simulink model "RB_KAIROS_ImpControl_OpSpace_quat_2020b_safety"  (R2020b)
settings: Solver=ode4  StartTime=0.0  StopTime=20  FixedStep=model_sample_time  RelTol=1e-3
values from neighbouring files (symbols this model uses):
  am = 0.3    [RB_KAIROS_ImpControl_OpSpace_quat_2020b_safety_main.m]
  am_r = 0.3    [RB_KAIROS_ImpControl_OpSpace_quat_2020b_safety_main.m]
  Kc = diag(50*ones(6,1))    [RB_KAIROS_ImpControl_OpSpace_quat_2020b_safety_main.m]
  Kp = 2*[400;400;400;400;0;0;0]    [RB_KAIROS_ImpControl_OpSpace_quat_2020b_safety_main.m]
  Kv = [1000;1000;1000;[300;300;300;300;300;300;300]]    [RB_KAIROS_ImpControl_OpSpace_quat_2020b_safety_main.m]
  model_sample_time = 0.001    [RB_KAIROS_ImpControl_OpSpace_quat_2020b_safety_main.m]
  q_dot_0 = zeros(10,1)    [RB_KAIROS_ImpControl_OpSpace_quat_2020b_safety_main.m]
  T_i = K    [RB_KAIROS_ImpControl_OpSpace_quat_2020b_safety_main.m]
  tau_ext = [0 0 0 0 0 0 0 0 0 0 0]    [RB_KAIROS_ImpControl_OpSpace_quat_2020b_safety_main.m]
  v_SMU = 10    [RB_KAIROS_ImpControl_OpSpace_quat_2020b_safety_main.m]
  vm = 0.5    [RB_KAIROS_ImpControl_OpSpace_quat_2020b_safety_main.m]
  vm_r = 0.5    [RB_KAIROS_ImpControl_OpSpace_quat_2020b_safety_main.m]
undefined symbols (not defined in the file or in its folder): DiscIntNeverNeededParam, magnitude, q_0, sigbuilder_block, T_f
libraries: simulink x4, utils x4, transformations_lib x3
(part 1 of 17)
settings Model: Creator=Alessandro  LastModifiedBy=ubuntu
settings DataIOCC: ReturnWorkspaceOutputs=off
settings DebuggingCC: UnconnectedInputMsg=none  UnconnectedOutputMsg=none  UnconnectedLineMsg=none  SFMachineParentedDataDiag=error
settings SFSimCC: SimUserIncludeDirs="\"/home/ubuntu/whole_body_control/whole-body-controller/Simulation/GeneratedFunctions/CppDynamics/include\""  SimTargetLang=C++
settings SFSimCC: SimCustomHeaderCode=|
  | #include "get_C.h"
  | #include "get_Cv.h"
  | #include "get_M.h"
  | #include "get_Mv.h"
  | #include "get_G.h"
settings SFSimCC: SimUserSources=|
  | "/home/ubuntu/whole_body_control/whole-body-controller/Simulation/GeneratedFunctions/CppDynamics/src/get_C.cpp"
  | "/home/ubuntu/whole_body_control/whole-body-controller/Simulation/GeneratedFunctions/CppDynamics/src/get_Cv.cpp"
  | "/home/ubuntu/whole_body_control/whole-body-controller/Simulation/GeneratedFunctions/CppDynamics/src/get_M.cpp"
  | "/home/ubuntu/whole_body_control/whole-body-controller/Simulation/GeneratedFunctions/CppDynamics/src/get_Mv.cpp"
  | "/home/ubuntu/whole_body_control/whole-body-controller/Simulation/GeneratedFunctions/CppDynamics/src/get_G.cpp"

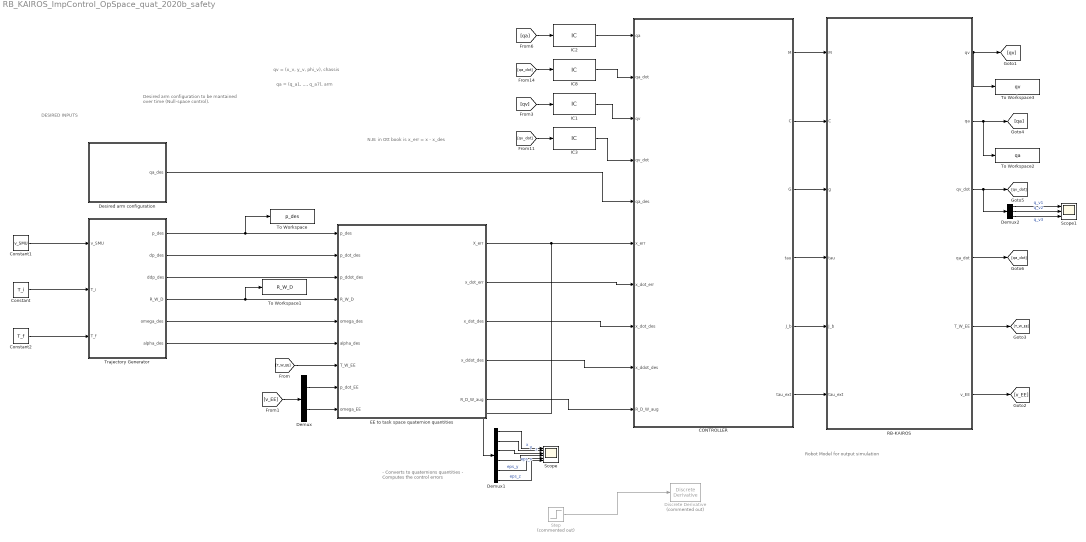
== system RB_KAIROS_ImpControl_OpSpace_quat_2020b_safety ==
  note: - Converts to quaternions quantities
      | - Computes the control errors
  note: Robot Model for output simulation
  note: DESIRED INPUTS
  note: N.B: in Ott book is x_err = x - x_des
  note: qv = (x_v, y_v, phi_v), chassis
  note: qa = (q_a1, ..., q_a7), arm
  note: Desired arm configuration to be mantained over time (Null-space control).
  "CONTROLLER " : Subsystem
  Constant : Constant  Value=T_i
  Constant1 : Constant  Value=v_SMU
  Constant2 : Constant  Value=T_f
  Demux : Demux  Outputs=2
  Demux1 : Demux  Outputs=6
  Demux2 : Demux  Outputs=3
  Desired arm configuration : Subsystem
  Discrete Derivative : simulink/Discrete/Discrete Derivative  Commented=on  gainval=1  ICPrevScaledInput=0.0  OutMin=[]  OutMax=[]  OutDataType=fixdt(1, 16)  OutScaling=2^-10  DoSatur=off
  EE to task space quaternion quantities : Subsystem
  IC1 : InitialCondition  Value=q_0([1:3])
  IC2 : InitialCondition  Value=q_0([4:10])
  IC3 : InitialCondition  Value=q_dot_0([1:3])
  IC8 : InitialCondition  Value=q_dot_0([4:10])
  RB-KAIROS : Subsystem
  Scope : Scope  NumInputPorts=6
  Scope1 : Scope  NumInputPorts=3
  Step : Step  Commented=on  Time=5  Before=zeros(10,1)  After=tau_ext  SampleTime=0
  To Workspace : ToWorkspace  VariableName=p_des  SaveFormat=Timeseries  SampleTime=-1
  To Workspace1 : ToWorkspace  VariableName=R_W_D  SaveFormat=Timeseries  SampleTime=-1
  To Workspace2 : ToWorkspace  VariableName=qa  SaveFormat=Timeseries  SampleTime=-1
      settings: Decimation=10
  To Workspace3 : ToWorkspace  VariableName=qv  SaveFormat=Timeseries  SampleTime=-1
      settings: Decimation=10
  Trajectory Generator : Subsystem
  wires:
  "CONTROLLER "/1(M) -> RB-KAIROS/1(M)
  RB-KAIROS/4(qa_dot) -> [qa_dot]
  RB-KAIROS/6(v_EE) -> [v_EE]
  "CONTROLLER "/3(G) -> RB-KAIROS/3(g)
  RB-KAIROS/2(qa) -> [qa], To Workspace2/1
  [qa_dot] -> IC8/1
  Desired arm configuration/1(qa_des) -> "CONTROLLER "/5(qa_des)
  [qv] -> IC1/1
  "CONTROLLER "/2(C) -> RB-KAIROS/2(C)
  RB-KAIROS/5(T_W_EE) -> [T_W_EE]
  [qv_dot] -> IC3/1
  "CONTROLLER "/4(tau) -> RB-KAIROS/4(tau)
  [qa] -> IC2/1
  RB-KAIROS/1(qv) -> [qv], To Workspace3/1
  [T_W_EE] -> EE to task space quaternion quantities/7(T_W_EE)
  "CONTROLLER "/5(J_b) -> RB-KAIROS/5(J_b)
  [v_EE] -> Demux/1
  Demux/2 -> EE to task space quaternion quantities/9(omega_EE)
  Demux/1 -> EE to task space quaternion quantities/8(p_dot_EE)
  EE to task space quaternion quantities/2(x_dot_err) -> "CONTROLLER "/7(x_dot_err)
  EE to task space quaternion quantities/3(x_dot_des) -> "CONTROLLER "/8(x_dot_des)
  EE to task space quaternion quantities/4(x_ddot_des) -> "CONTROLLER "/9(x_ddot_des)
  EE to task space quaternion quantities/5(R_D_W_aug) -> "CONTROLLER "/10(R_D_W_aug)
  IC2/1 -> "CONTROLLER "/1(qa)
  IC8/1 -> "CONTROLLER "/2(qa_dot)
  IC1/1 -> "CONTROLLER "/3(qv)
  IC3/1 -> "CONTROLLER "/4(qv_dot)
  Constant1/1 -> Trajectory Generator/1(v_SMU)
  Constant/1 -> Trajectory Generator/2(T_i)
  Constant2/1 -> Trajectory Generator/3(T_f)
  Trajectory Generator/1(p_des) -> To Workspace/1, EE to task space quaternion quantities/1(p_des)
  Trajectory Generator/2(dp_des) -> EE to task space quaternion quantities/2(p_dot_des)
  Trajectory Generator/3(ddp_des) -> EE to task space quaternion quantities/3(p_ddot_des)
  Trajectory Generator/5(omega_des) -> EE to task space quaternion quantities/5(omega_des)
  Trajectory Generator/6(alpha_des) -> EE to task space quaternion quantities/6(alpha_des)
  Trajectory Generator/4(R_W_D) -> To Workspace1/1, EE to task space quaternion quantities/4(R_W_D)
  EE to task space quaternion quantities/1(X_err) -> Demux1/1, "CONTROLLER "/6(x_err)
  Demux1/6 -> Scope/6  "eps_z"
  Demux1/4 -> Scope/4  "eps_x"
  Demux1/2 -> Scope/2  "y"
  Demux1/5 -> Scope/5  "eps_y"
  Demux1/3 -> Scope/3  "z"
  Demux1/1 -> Scope/1  "x"
  Demux2/3 -> Scope1/3  "q_v3"
  RB-KAIROS/3(qv_dot) -> Demux2/1, [qv_dot]
  Demux2/2 -> Scope1/2  "q_v2"
  Demux2/1 -> Scope1/1  "q_v1"
  Step/1 -> Discrete Derivative/1
  "CONTROLLER "/6(tau_ext) -> RB-KAIROS/6(tau_ext)

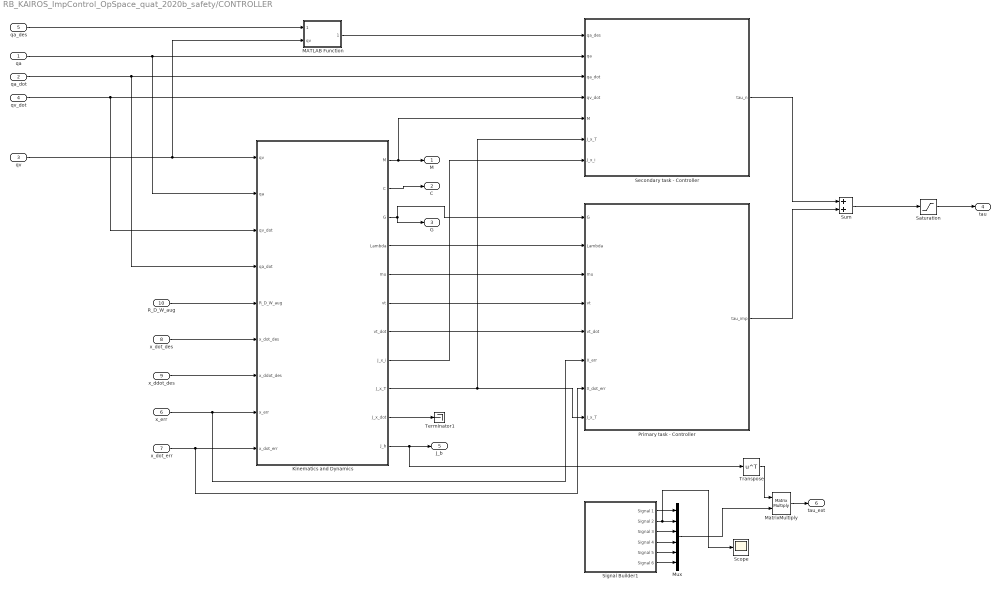
== system RB_KAIROS_ImpControl_OpSpace_quat_2020b_safety/CONTROLLER  ==
  qa : Inport
  qa_dot : Inport  Port=2
  qv : Inport  Port=3
  qv_dot : Inport  Port=4
  qa_des : Inport  Port=5
  x_err : Inport  Port=6
  x_dot_err : Inport  Port=7
  x_dot_des : Inport  Port=8
  x_ddot_des : Inport  Port=9
  R_D_W_aug : Inport  Port=10
  Kinematics and Dynamics : Subsystem
  MATLAB Function : MATLAB Function  TreatAsAtomicUnit=on
  MatrixMultiply : Product  Multiplication=Matrix(*)
  Mux : Mux  Inputs=6
  Primary task - Controller : Subsystem
  Saturation : Saturate  UpperLimit=|  LowerLimit=|
      UpperLimit=|
      | [[300; 300; 300]; 87;
      | 87;
      | 87;
      | 87;
      | 12;
      | 12; 12]
      LowerLimit=|
      | -[[300; 300; 300]; 87;
      | 87;
      | 87;
      | 87;
      | 12;
      | 12; 12]
  Scope : Scope
  Secondary task - Controller : Subsystem
  Signal Builder1 : Subsystem  Tag=STV Subsys  LoadFcn=sigbuilder_block('load',[721.5 -243.75 1378.5 558.75 ]);  StartFcn=sigbuilder_block('start');  StopFcn=sigbuilder_block('stop');  ClipboardFcn=sigbuilder_block('clipboard');  mask(Sigbuilder block){tuvar=[0:10]}
      mask help: Simulink:masks:SigbuilderBlock_MD
      mask init:
      | if ~strcmp(get_param(bdroot(gcbh),'SimulationStatus'),'stopped') tuvar = sigbuilder_block('maskInit'); end
      settings: CopyFcn=sigbuilder_block('copy');  DeleteFcn=sigbuilder_block('delete');  ModelCloseFcn=sigbuilder_block('modelClose');  PreSaveFcn=sigbuilder_block('preSave');  PauseFcn=sigbuilder_block('pause');  ContinueFcn=sigbuilder_block('continue');  NameChangeFcn=sigbuilder_block('namechange');  OpenFcn=sigbuilder_block('open',[-114 -87.75 1386 594 ]);  CloseFcn=sigbuilder_block('close');
      mask Display: plot(0, 0, 100, 100,[2, 2, 32, 32, 2], [68, 8, 8, 68, 68],[32, 2], [38, 38], [32, 19, 2],[53, 60, 44], [32, 17, 17, 2],[16, 16, 31, 31]);txt = getActiveGroup(gcbh);text(2, 100, txt,'verticalAlignment', 'top');
  Sum : Sum
  Terminator1 : Terminator
  Transpose : Math  Operator=transpose  SaturateOnIntegerOverflow=on
  M : Outport
  C : Outport  Port=2
  G : Outport  Port=3
  tau : Outport  Port=4
  J_b : Outport  Port=5
  tau_ext : Outport  Port=6
  wires:
  qv_dot/1 -> Secondary task - Controller/4(qv_dot), Kinematics and Dynamics/3(qv_dot)
  Primary task - Controller/1(tau_imp) -> Sum/2
  qv/1 -> Kinematics and Dynamics/1(qv), MATLAB Function/2(qv)
  qa/1 -> Secondary task - Controller/2(qa), Kinematics and Dynamics/2(qa)
  qa_dot/1 -> Kinematics and Dynamics/4(qa_dot), Secondary task - Controller/3(qa_dot)
  Kinematics and Dynamics/9(J_x_T) -> Primary task - Controller/8(J_x_T), Secondary task - Controller/6(J_x_T)
  Kinematics and Dynamics/8(J_x_i) -> Secondary task - Controller/7(J_x_i)
  Secondary task - Controller/1(tau_n) -> Sum/1
  Kinematics and Dynamics/3(G) -> Primary task - Controller/1(G), G/1
  Sum/1 -> Saturation/1
  Kinematics and Dynamics/1(M) -> M/1, Secondary task - Controller/5(M)
  qa_des/1 -> MATLAB Function/1(qa_des)
  Kinematics and Dynamics/2(C) -> C/1
  Saturation/1 -> tau/1
  R_D_W_aug/1 -> Kinematics and Dynamics/5(R_D_W_aug)
  x_dot_des/1 -> Kinematics and Dynamics/6(x_dot_des)
  x_ddot_des/1 -> Kinematics and Dynamics/7(x_ddot_des)
  x_dot_err/1 -> Primary task - Controller/7(X_dot_err), Kinematics and Dynamics/9(x_dot_err)
  Kinematics and Dynamics/6(vt) -> Primary task - Controller/4(vt)
  Kinematics and Dynamics/7(vt_dot) -> Primary task - Controller/5(vt_dot)
  Kinematics and Dynamics/11(J_b) -> Transpose/1, J_b/1
  Kinematics and Dynamics/10(J_x_dot) -> Terminator1/1
  Kinematics and Dynamics/4(Lambda) -> Primary task - Controller/2(Lambda)
  Kinematics and Dynamics/5(mu) -> Primary task - Controller/3(mu)
  MATLAB Function/1(qa_des_new) -> Secondary task - Controller/1(qa_des)
  x_err/1 -> Kinematics and Dynamics/8(x_err), Primary task - Controller/6(X_err)
  MatrixMultiply/1 -> tau_ext/1
  Transpose/1 -> MatrixMultiply/1
  Mux/1 -> MatrixMultiply/2
  Signal Builder1/5(Signal 5) -> Mux/5
  Signal Builder1/1(Signal 1) -> Mux/1
  Signal Builder1/3(Signal 3) -> Mux/3
  Signal Builder1/6(Signal 6) -> Mux/6
  Signal Builder1/4(Signal 4) -> Mux/4
  Signal Builder1/2(Signal 2) -> Scope/1, Mux/2

== system RB_KAIROS_ImpControl_OpSpace_quat_2020b_safety/Desired arm configuration ==
  Constant : Constant  Value=[0, -0.785, 0, -2.356, 0, 1.57, 0.785]'  SampleTime=model_sample_time
  qa_des : Outport
  wires:
  Constant/1 -> qa_des/1

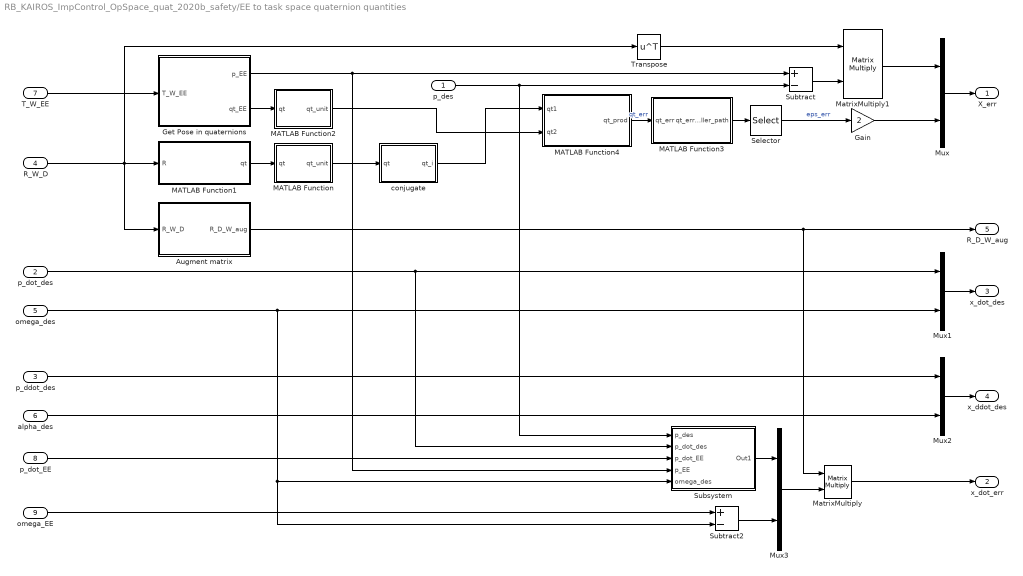
== system RB_KAIROS_ImpControl_OpSpace_quat_2020b_safety/EE to task space quaternion quantities ==
  p_des : Inport
  p_dot_des : Inport  Port=2
  p_ddot_des : Inport  Port=3
  R_W_D : Inport  Port=4
  omega_des : Inport  Port=5
  alpha_des : Inport  Port=6
  T_W_EE : Inport  Port=7
  p_dot_EE : Inport  Port=8
  omega_EE : Inport  Port=9
  Augment matrix : MATLAB Function  TreatAsAtomicUnit=on
  Gain : Gain  Gain=2
  Get Pose in quaternions : MATLAB Function  TreatAsAtomicUnit=on
  MATLAB Function : MATLAB Function  TreatAsAtomicUnit=on
  MATLAB Function1 : MATLAB Function  TreatAsAtomicUnit=on
  MATLAB Function2 : MATLAB Function  TreatAsAtomicUnit=on
  MATLAB Function3 : MATLAB Function  TreatAsAtomicUnit=on
  MATLAB Function4 : MATLAB Function  TreatAsAtomicUnit=on
  MatrixMultiply : Product  Multiplication=Matrix(*)
  MatrixMultiply1 : Product  Multiplication=Matrix(*)
  Mux{,1..3} (4 alike) : Mux  Inputs=2
  Selector : Selector  InputPortWidth=4  IndexOptions=Index vector (dialog)  Indices=[2:4]  OutputSizes=1
  Subsystem : Subsystem
  Subtract : Sum  Inputs=+-
  Subtract2 : Sum  Inputs=+-
  Transpose : Math  Operator=transpose  SaturateOnIntegerOverflow=on
  conjugate : MATLAB Function  TreatAsAtomicUnit=on
  X_err : Outport
  x_dot_err : Outport  Port=2
  x_dot_des : Outport  Port=3
  x_ddot_des : Outport  Port=4
  R_D_W_aug : Outport  Port=5
  wires:
  Get Pose in quaternions/1(p_EE) -> Subtract/1, Subsystem/4(p_EE)
  Subtract/1 -> MatrixMultiply1/2
  p_des/1 -> Subtract/2, Subsystem/1(p_des)
  T_W_EE/1 -> Get Pose in quaternions/1(T_W_EE)
  MATLAB Function4/1(qt_prod) -> MATLAB Function3/1(qt_err)  "qt_err"
  R_W_D/1 -> MATLAB Function1/1(R), Transpose/1, Augment matrix/1(R_W_D)
  Mux/1 -> X_err/1
  MATLAB Function1/1(qt) -> MATLAB Function/1(qt)
  p_dot_des/1 -> Mux1/1, Subsystem/2(p_dot_des)
  Get Pose in quaternions/2(qt_EE) -> MATLAB Function2/1(qt)
  Selector/1 -> Gain/1  "eps_err"
  Augment matrix/1(R_D_W_aug) -> R_D_W_aug/1, MatrixMultiply/1
  omega_des/1 -> Mux1/2, Subsystem/5(omega_des), Subtract2/2
  Mux1/1 -> x_dot_des/1
  Mux2/1 -> x_ddot_des/1
  alpha_des/1 -> Mux2/2
  p_ddot_des/1 -> Mux2/1
  omega_EE/1 -> Subtract2/1
  Subtract2/1 -> Mux3/2
  Mux3/1 -> MatrixMultiply/2
  MatrixMultiply/1 -> x_dot_err/1
  MatrixMultiply1/1 -> Mux/1
  Gain/1 -> Mux/2
  p_dot_EE/1 -> Subsystem/3(p_dot_EE)
  Subsystem/1(Out1) -> Mux3/1
  MATLAB Function/1(qt_unit) -> conjugate/1(qt)
  MATLAB Function2/1(qt_unit) -> MATLAB Function4/2(qt2)
  conjugate/1(qt_i) -> MATLAB Function4/1(qt1)
  Transpose/1 -> MatrixMultiply1/1
  MATLAB Function3/1(qt_err_smaller_path) -> Selector/1

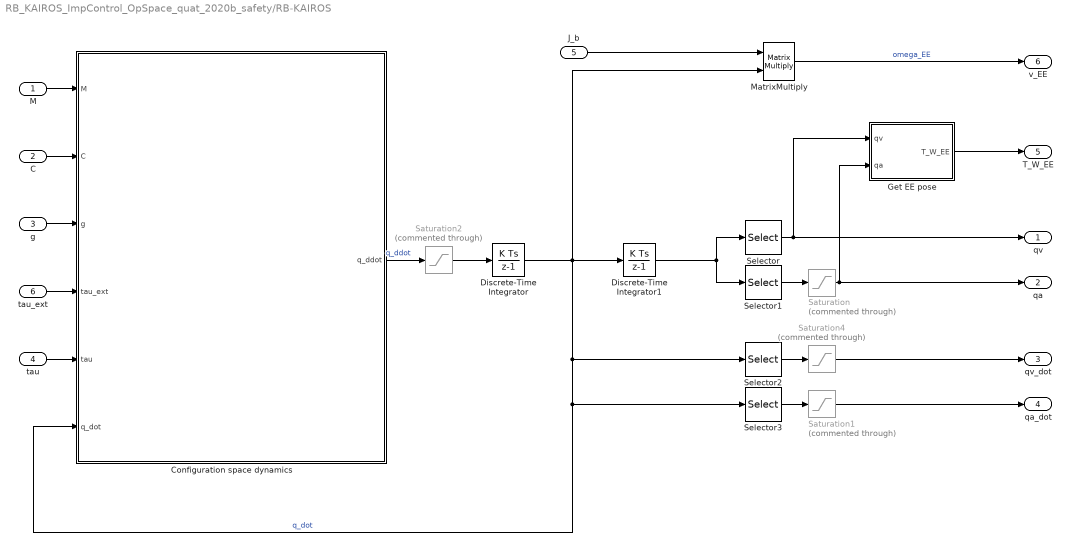
== system RB_KAIROS_ImpControl_OpSpace_quat_2020b_safety/RB-KAIROS ==
  M : Inport
  C : Inport  Port=2
  g : Inport  Port=3
  tau : Inport  Port=4
  J_b : Inport  Port=5
  tau_ext : Inport  Port=6
  Configuration space dynamics : MATLAB Function  TreatAsAtomicUnit=on
  Discrete-Time Integrator : DiscreteIntegrator  InitialCondition=q_dot_0  SampleTime=model_sample_time  ICPrevOutput=DiscIntNeverNeededParam  ICPrevScaledInput=DiscIntNeverNeededParam
  Discrete-Time Integrator1 : DiscreteIntegrator  InitialCondition=q_0  SampleTime=model_sample_time  ICPrevOutput=DiscIntNeverNeededParam  ICPrevScaledInput=DiscIntNeverNeededParam
  Get EE pose : Subsystem
  MatrixMultiply : Product  Multiplication=Matrix(*)
  Saturation : Saturate  Commented=through  UpperLimit=[2.3093; 1.5133; 2.4937; -0.4461; 2.4800; 4.2094; 2.6895]  LowerLimit=[-2.3093; -1.5133; -2.4937; -2.7478; -2.4800; 0.8521; -2.6895]
  Saturation1 : Saturate  Commented=through  UpperLimit=[2; 1; 1.5; 1.25; 3; 1.5; 3]  LowerLimit=-[2; 1; 1.5; 1.25; 3; 1.5; 3]
  Saturation2 : Saturate  Commented=through  UpperLimit=|  LowerLimit=|
      UpperLimit=|
      | [20*ones(3,1); 15;
      | 7.5;
      | 10;
      | 12.5;
      | 15;
      | 20;
      | 20;]
      LowerLimit=|
      | -[20*ones(3,1); 15;
      | 7.5;
      | 10;
      | 12.5;
      | 15;
      | 20;
      | 20;]
  Saturation4 : Saturate  Commented=through  UpperLimit=1*ones(3,1)  LowerLimit=-1*ones(3,1)
  Selector : Selector  IndexOptions=Index vector (dialog)  Indices=[1:3]  OutputSizes=1
  Selector1 : Selector  IndexOptions=Index vector (dialog)  Indices=[4:10]  OutputSizes=1
  Selector2 : Selector  IndexOptions=Index vector (dialog)  Indices=[1:3]  OutputSizes=1
  Selector3 : Selector  IndexOptions=Index vector (dialog)  Indices=[4:10]  OutputSizes=1
  qv : Outport
  qa : Outport  Port=2
  qv_dot : Outport  Port=3
  qa_dot : Outport  Port=4
  T_W_EE : Outport  Port=5
  v_EE : Outport  Port=6
  wires:
  M/1 -> Configuration space dynamics/1(M)
  C/1 -> Configuration space dynamics/2(C)
  g/1 -> Configuration space dynamics/3(g)
  tau/1 -> Configuration space dynamics/5(tau)
  tau_ext/1 -> Configuration space dynamics/4(tau_ext)
  Configuration space dynamics/1(q_ddot) -> Saturation2/1  "q_ddot"
  Selector1/1 -> Saturation/1
  Saturation/1 -> Get EE pose/2(qa), qa/1
  Discrete-Time Integrator1/1 -> Selector/1, Selector1/1
  Selector/1 -> Get EE pose/1(qv), qv/1
  Saturation4/1 -> qv_dot/1
  Saturation1/1 -> qa_dot/1
  Selector2/1 -> Saturation4/1
  Discrete-Time Integrator/1 -> Discrete-Time Integrator1/1, MatrixMultiply/2, Configuration space dynamics/6(q_dot), Selector3/1, Selector2/1  "q_dot"
  Selector3/1 -> Saturation1/1
  MatrixMultiply/1 -> v_EE/1  "omega_EE"
  Saturation2/1 -> Discrete-Time Integrator/1
  Get EE pose/1(T_W_EE) -> T_W_EE/1
  J_b/1 -> MatrixMultiply/1

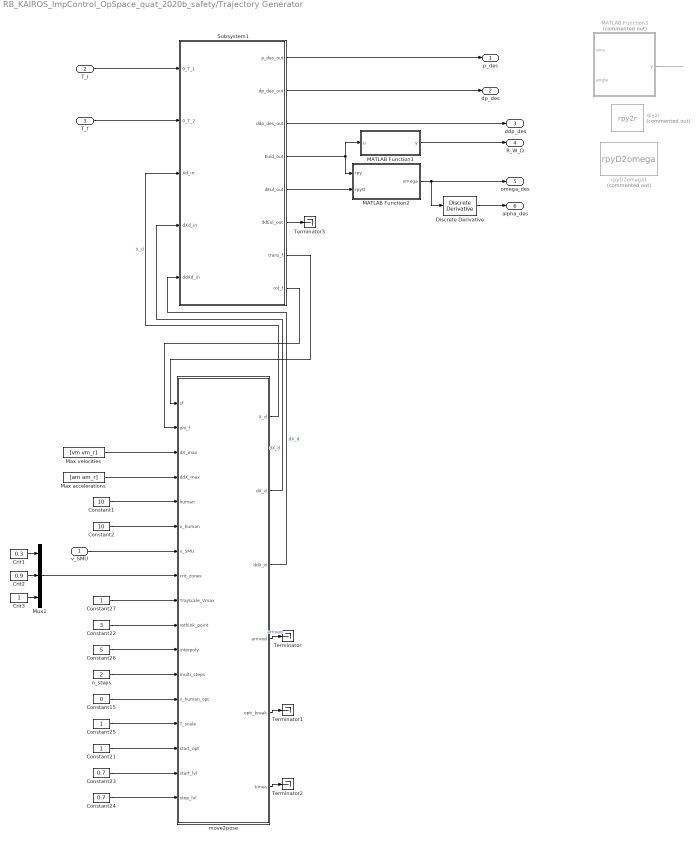
== system RB_KAIROS_ImpControl_OpSpace_quat_2020b_safety/Trajectory Generator ==
  v_SMU : Inport
  T_i : Inport  Port=2
  T_f : Inport  Port=3
  Constant1 : Constant  Value=10
  Constant15 : Constant  Value=0
  Constant2 : Constant  Value=10
  Constant21 : Constant
  Constant22 : Constant  Value=3
  Constant23 : Constant  Value=0.7
  Constant24 : Constant  Value=0.7
  Constant25 : Constant
  Constant26 : Constant  Value=5
  Constant27 : Constant
  Crit1 : Constant  Value=0.3
  Crit2 : Constant  Value=0.9
  Crit3 : Constant
  Discrete Derivative : simulink/Discrete/Discrete Derivative  gainval=1.0  ICPrevScaledInput=0.0  OutMin=[]  OutMax=[]  OutDataType=fixdt(1, 16)  OutScaling=2^-10  DoSatur=off
  MATLAB Function1 : MATLAB Function  TreatAsAtomicUnit=on
  MATLAB Function2 : MATLAB Function  TreatAsAtomicUnit=on
  MATLAB Function3 : MATLAB Function  Commented=on  TreatAsAtomicUnit=on
  Max accelerations : Constant  Value=[am am_r]
  Max velocities : Constant  Value=[vm vm_r]
  Mux1 : Mux  Inputs=3
  Subsystem1 : Subsystem
  Terminator{,1..3} (4 alike) : Terminator
  move2pose : Subsystem
  n_steps : Constant  Value=2
  rpy2r : transformations_lib/rpy2r  Commented=on  SystemSampleTime=-1  VariantActivationTime=update diagram  Latency=0  AutoFrameSizeCalculation=off
  rpyD2omega1 : transformations_lib/rpyD2omega  Commented=on  SystemSampleTime=-1  VariantActivationTime=update diagram  Latency=0  AutoFrameSizeCalculation=off
  p_des : Outport
  dp_des : Outport  Port=2
  ddp_des : Outport  Port=3
  R_W_D : Outport  Port=4
  omega_des : Outport  Port=5
  alpha_des : Outport  Port=6
  wires:
  move2pose/1(X_d) -> Subsystem1/3(Xd_in)  "X_d"
  move2pose/2(dX_d) -> Subsystem1/4(dXd_in)  "dX_d"
  move2pose/3(ddX_d) -> Subsystem1/5(ddXd_in)  "dX_d"
  Max velocities/1 -> move2pose/3(dX_max)
  Max accelerations/1 -> move2pose/4(ddX_max)
  v_SMU/1 -> move2pose/7(v_SMU)
  Crit3/1 -> Mux1/3
  Crit2/1 -> Mux1/2
  Crit1/1 -> Mux1/1
  Mux1/1 -> move2pose/8(crit_zones)
  Constant25/1 -> move2pose/14(T_scale)
  Constant27/1 -> move2pose/9(TrajScale_Vmax)
  n_steps/1 -> move2pose/12(multi_steps)
  Constant21/1 -> move2pose/15(start_opt)
  Constant22/1 -> move2pose/10(rethink_point)
  Constant23/1 -> move2pose/16(start_lvl)
  Constant15/1 -> move2pose/13(v_human_opt)
  Constant24/1 -> move2pose/17(stop_lvl)
  Constant26/1 -> move2pose/11(interpoly)
  Subsystem1/4(Euld_out) -> MATLAB Function1/1(u), MATLAB Function2/1(rpy)
  Subsystem1/1(p_des_out) -> p_des/1
  Subsystem1/3(ddp_des_out) -> ddp_des/1
  Subsystem1/2(dp_des_out) -> dp_des/1
  Subsystem1/7(trans_f) -> move2pose/1(sf)
  Subsystem1/8(rot_f) -> move2pose/2(phi_f)
  move2pose/6(times) -> Terminator2/1
  move2pose/5(opti_break) -> Terminator1/1
  move2pose/4(arrived) -> Terminator/1  "arrived"
  T_i/1 -> Subsystem1/1(0_T_1)
  T_f/1 -> Subsystem1/2(0_T_2)
  MATLAB Function1/1(y) -> R_W_D/1
  MATLAB Function2/1(omega) -> omega_des/1, Discrete Derivative/1
  Constant1/1 -> move2pose/5(human)
  Constant2/1 -> move2pose/6(v_human)
  MATLAB Function3/1(y) -> ?
  Subsystem1/5(dEul_out) -> MATLAB Function2/2(rpyD)
  Discrete Derivative/1 -> alpha_des/1
  Subsystem1/6(ddEul_out) -> Terminator3/1

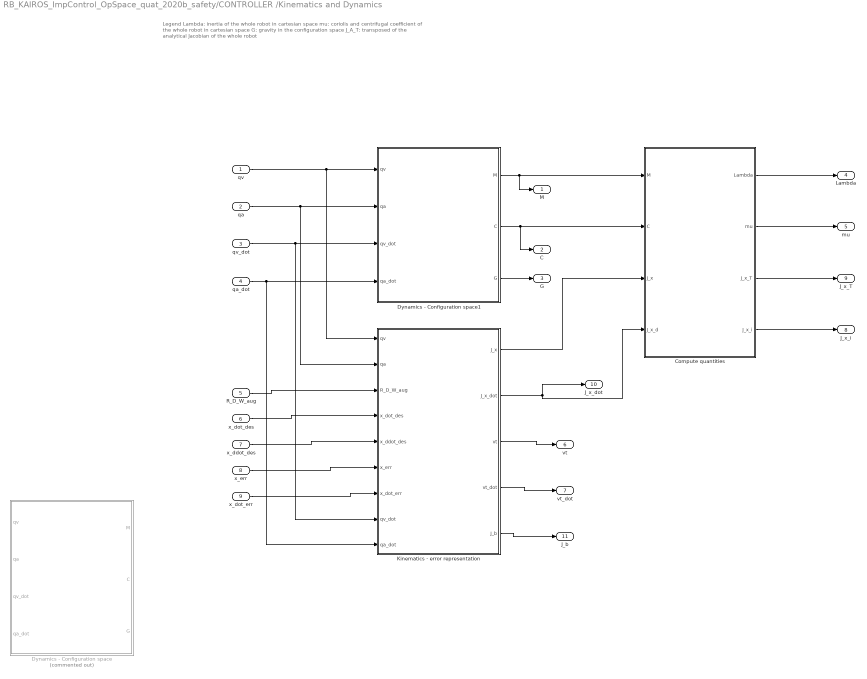
== system RB_KAIROS_ImpControl_OpSpace_quat_2020b_safety/CONTROLLER /Kinematics and Dynamics ==
  note: Legend
      | Lambda: inertia of the whole robot in cartesian space
      | mu: coriolis and centrifugal coefficient of the whole robot in cartesian space
      | G: gravity in the configuration space
      | J_A_T: transposed of the analytical Jacobian of the whole robot
  qv : Inport
  qa : Inport  Port=2
  qv_dot : Inport  Port=3
  qa_dot : Inport  Port=4
  R_D_W_aug : Inport  Port=5
  x_dot_des : Inport  Port=6
  x_ddot_des : Inport  Port=7
  x_err : Inport  Port=8
  x_dot_err : Inport  Port=9
  Compute quantities : MATLAB Function  TreatAsAtomicUnit=on
  Dynamics - Configuration space : Subsystem  Commented=on
  Dynamics - Configuration space1 : Subsystem
  Kinematics - error representation : Subsystem
  M : Outport
  C : Outport  Port=2
  G : Outport  Port=3
  Lambda : Outport  Port=4
  mu : Outport  Port=5
  vt : Outport  Port=6
  vt_dot : Outport  Port=7
  J_x_i : Outport  Port=8
  J_x_T : Outport  Port=9
  J_x_dot : Outport  Port=10
  J_b : Outport  Port=11
  wires:
  Compute quantities/1(Lambda) -> Lambda/1
  Compute quantities/2(mu) -> mu/1
  qv/1 -> Dynamics - Configuration space1/1(qv), Kinematics - error representation/1(qv)
  qa/1 -> Kinematics - error representation/2(qa), Dynamics - Configuration space1/2(qa)
  qv_dot/1 -> Kinematics - error representation/8(qv_dot), Dynamics - Configuration space1/3("qv_dot ")
  Dynamics - Configuration space1/1(M) -> M/1, Compute quantities/1(M)
  Dynamics - Configuration space1/2(C) -> C/1, Compute quantities/2(C)
  Dynamics - Configuration space1/3(G) -> G/1
  Compute quantities/3(J_x_T) -> J_x_T/1
  Compute quantities/4(J_x_i) -> J_x_i/1
  Kinematics - error representation/1(J_x) -> Compute quantities/3(J_x)
  Kinematics - error representation/2(J_x_dot) -> Compute quantities/4(J_x_d), J_x_dot/1
  Kinematics - error representation/3(vt) -> vt/1
  Kinematics - error representation/4(vt_dot) -> vt_dot/1
  R_D_W_aug/1 -> Kinematics - error representation/3(R_D_W_aug)
  x_dot_des/1 -> Kinematics - error representation/4(x_dot_des)
  x_ddot_des/1 -> Kinematics - error representation/5(x_ddot_des)
  Kinematics - error representation/5(J_b) -> J_b/1
  x_err/1 -> Kinematics - error representation/6(x_err)
  x_dot_err/1 -> Kinematics - error representation/7(x_dot_err)
  qa_dot/1 -> Kinematics - error representation/9(qa_dot), Dynamics - Configuration space1/4(qa_dot)

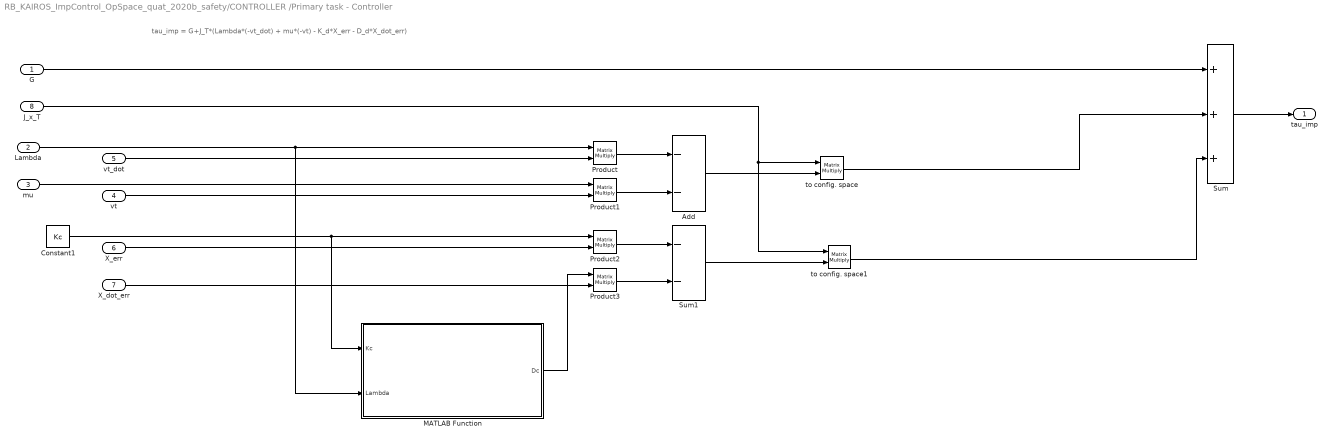
== system RB_KAIROS_ImpControl_OpSpace_quat_2020b_safety/CONTROLLER /Primary task - Controller ==
  note: tau_imp = G+J_T*(Lambda*(-vt_dot) + mu*(-vt) - K_d*X_err - D_d*X_dot_err)
  G : Inport
  Lambda : Inport  Port=2
  mu : Inport  Port=3
  vt : Inport  Port=4
  vt_dot : Inport  Port=5
  X_err : Inport  Port=6
  X_dot_err : Inport  Port=7
  J_x_T : Inport  Port=8
  Add : Sum  Inputs=--
  Constant1 : Constant  Value=Kc
  MATLAB Function : MATLAB Function  TreatAsAtomicUnit=on
  Product{,1..3} (4 alike) : Product  Multiplication=Matrix(*)
  Sum : Sum  Inputs=+++
  Sum1 : Sum  Inputs=--
  to config. space : Product  Multiplication=Matrix(*)
  to config. space1 : Product  Multiplication=Matrix(*)
  tau_imp : Outport
  wires:
  mu/1 -> Product1/1
  Product2/1 -> Sum1/1
  vt_dot/1 -> Product/2
  vt/1 -> Product1/2
  Product3/1 -> Sum1/2
  Lambda/1 -> Product/1, MATLAB Function/2(Lambda)
  to config. space/1 -> Sum/2
  X_err/1 -> Product2/2
  X_dot_err/1 -> Product3/2
  G/1 -> Sum/1
  Product1/1 -> Add/2
  Product/1 -> Add/1
  Add/1 -> to config. space/2
  Sum/1 -> tau_imp/1
  Sum1/1 -> to config. space1/2
  J_x_T/1 -> to config. space/1, to config. space1/1
  MATLAB Function/1(Dc) -> Product3/1
  Constant1/1 -> Product2/1, MATLAB Function/1(Kc)
  to config. space1/1 -> Sum/3

== system RB_KAIROS_ImpControl_OpSpace_quat_2020b_safety/CONTROLLER /Secondary task - Controller ==
  qa_des : Inport
  qa : Inport  Port=2
  qa_dot : Inport  Port=3
  qv_dot : Inport  Port=4
  M : Inport  Port=5
  J_x_T : Inport  Port=6
  J_x_i : Inport  Port=7
  Constant : Constant  Value=Kp
  Constant1 : Constant  Value=Kv
  MATLAB Function : MATLAB Function  TreatAsAtomicUnit=on
  tau_n : Outport
  wires:
  qa/1 -> MATLAB Function/2(qa)
  qa_des/1 -> MATLAB Function/1(qa_des)
  M/1 -> MATLAB Function/5(M)
  qa_dot/1 -> MATLAB Function/3(qa_dot)
  MATLAB Function/1(tau_n) -> tau_n/1
  qv_dot/1 -> MATLAB Function/4(qv_dot)
  J_x_T/1 -> MATLAB Function/6(J_x_T)
  J_x_i/1 -> MATLAB Function/7(J_x_i)
  Constant/1 -> MATLAB Function/8(Kp)
  Constant1/1 -> MATLAB Function/9(Kv)

== system RB_KAIROS_ImpControl_OpSpace_quat_2020b_safety/CONTROLLER /Signal Builder1 ==
  Demux : Demux  Tag=STV Demux  Outputs=6
      settings: DisplayOption=none
  FromWs : FromWorkspace  Tag=STV FromWs  VariableName=tuvar  OutputAfterFinalValue=Setting to zero
      SigBuilderData=|
      | common.afterFinalStr = 'Set to zero'
      | common.sampleTime = '0'
      | dataSet.timeRange = [0 7]
      | dataSet.name = 'Group 1'
      | sbobj.Groups.Name = 'Group 1'
      | sbobj.Groups.Signals(1).Name = 'Signal 1'
      | sbobj.Groups.Signals(1).XData = [0 7]
      | sbobj.Groups.Signals(1).YData = [0 0]
      | sbobj.Groups.Signals(2).Name = 'Signal 2'
      | sbobj.Groups.Signals(2).XData = [0 3 4 6 7]
      | sbobj.Groups.Signals(2).YData = [0 0 100 100 0]
      | sbobj.Groups.Signals(3).Name = 'Signal 3'
      | sbobj.Groups.Signals(3).XData = [0 7]
      | sbobj.Groups.Signals(3).YData = [0 0]
      | sbobj.Groups.Signals(4).Name = 'Signal 4'
      | sbobj.Groups.Signals(4).XData = [0 7]
      | sbobj.Groups.Signals(4).YData = [0 0]
      | sbobj.Groups.Signals(5).Name = 'Signal 5'
      | sbobj.Groups.Signals(5).XData = [0 7]
      | sbobj.Groups.Signals(5).YData = [0 0]
      | sbobj.Groups.Signals(6).Name = 'Signal 6'
      | sbobj.Groups.Signals(6).XData = [0 7]
      | sbobj.Groups.Signals(6).YData = [0 0]
      | sbobj.Groups.TimeRange = [0 7]
  Signal 1 : Outport  Tag=STV Outport
  Signal 2 : Outport  Tag=STV Outport  Port=2
  Signal 3 : Outport  Tag=STV Outport  Port=3
  Signal 4 : Outport  Tag=STV Outport  Port=4
  Signal 5 : Outport  Tag=STV Outport  Port=5
  Signal 6 : Outport  Tag=STV Outport  Port=6
  wires:
  FromWs/1 -> Demux/1
  Demux/1 -> Signal 1/1
  Demux/2 -> Signal 2/1
  Demux/3 -> Signal 3/1
  Demux/4 -> Signal 4/1
  Demux/5 -> Signal 5/1
  Demux/6 -> Signal 6/1

== system RB_KAIROS_ImpControl_OpSpace_quat_2020b_safety/EE to task space quaternion quantities/Subsystem ==
  p_des : Inport
  p_dot_des : Inport  Port=2
  p_dot_EE : Inport  Port=3
  p_EE : Inport  Port=4
  omega_des : Inport  Port=5
  Add : Sum  Inputs=+-
  MatrixMultiply : Product  Multiplication=Matrix(*)
  S(omega) : MATLAB Function  TreatAsAtomicUnit=on
  Subtract1 : Sum  Inputs=+--
  Out1 : Outport
  wires:
  Subtract1/1 -> Out1/1
  p_dot_EE/1 -> Subtract1/1
  p_dot_des/1 -> Subtract1/2
  omega_des/1 -> S(omega)/1(v)
  S(omega)/1(S) -> MatrixMultiply/1
  p_EE/1 -> Add/1
  p_des/1 -> Add/2
  Add/1 -> MatrixMultiply/2
  MatrixMultiply/1 -> Subtract1/3

== system RB_KAIROS_ImpControl_OpSpace_quat_2020b_safety/RB-KAIROS/Get EE pose ==
  qv : Inport
  qa : Inport  Port=2
  MATLAB Function : MATLAB Function  TreatAsAtomicUnit=on
  get_T_A_EE : MATLAB Function  TreatAsAtomicUnit=on
  T_W_EE : Outport
  wires:
  get_T_A_EE/1(T_A_EE) -> MATLAB Function/1(T_A_EE)
  MATLAB Function/1(T_W_EE) -> T_W_EE/1
  qa/1 -> get_T_A_EE/2(qa)
  qv/1 -> MATLAB Function/2(qv), get_T_A_EE/1(qv)

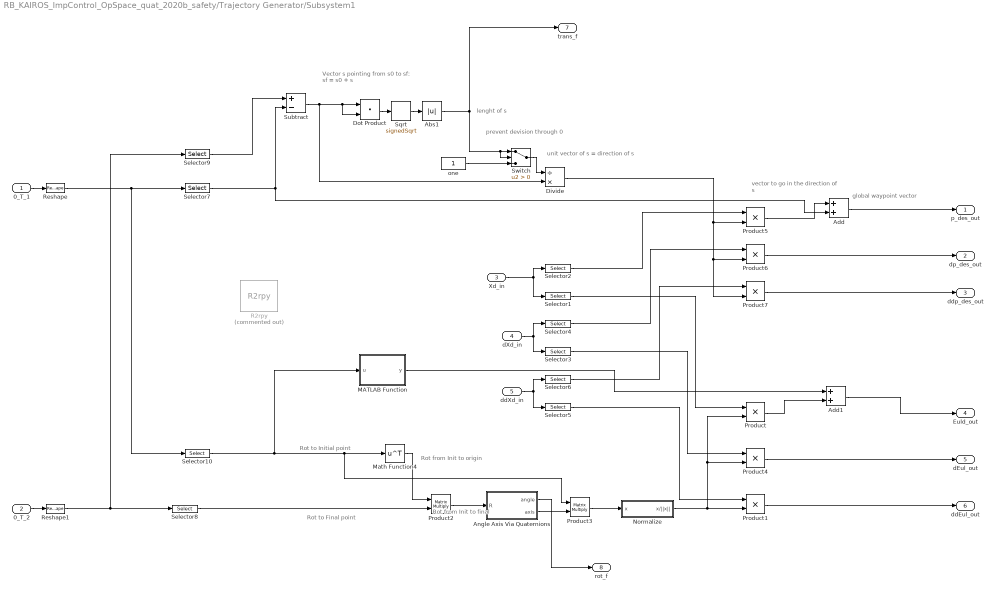
== system RB_KAIROS_ImpControl_OpSpace_quat_2020b_safety/Trajectory Generator/Subsystem1 ==
  note: Rot to Final point
  note: Rot to Initial point
  note: Rot from
      | Init to final
  note: Rot from Init to origin
  note: lenght of s
  note: vector to go in
      | the direction of s
  note: unit vector of s
      | = direction of s
  note: global waypoint vector
  note: prevent devision
      | through 0
  note: Vector s pointing
      | from s0 to sf:
      |  sf = s0 + s
  0_T_1 : Inport
  0_T_2 : Inport  Port=2
  Xd_in : Inport  Port=3
  dXd_in : Inport  Port=4
  ddXd_in : Inport  Port=5
  Abs1 : Abs
  Add : Sum
  Add1 : Sum
  Angle Axis Via Quaternions : Subsystem
  Divide : Product  Inputs=/*
  Dot Product : DotProduct  OutMin=0  InputSameDT=on  OutDataTypeStr=Inherit: Inherit via internal rule
  MATLAB Function : MATLAB Function  TreatAsAtomicUnit=on
  Math Function4 : Math  Operator=transpose  SignedPower=on  SaturateOnIntegerOverflow=on
  Normalize : Subsystem
  Product{,1,4..7} (6 alike) : Product
  Product2 : Product  Multiplication=Matrix(*)  RndMeth=Zero
  Product3 : Product  Multiplication=Matrix(*)
  R2rpy : transformations_lib/R2rpy  Commented=on  SystemSampleTime=-1  VariantActivationTime=update diagram  Latency=0  AutoFrameSizeCalculation=off
  Reshape : Reshape  OutputDimensionality=Customize  OutputDimensions=[4,4]
  Reshape1 : Reshape  OutputDimensionality=Customize  OutputDimensions=[4,4]
  Selector1 : Selector  InputPortWidth=2  IndexOptions=Index vector (dialog)  Indices=2  OutputSizes=1
  Selector10 : Selector  NumberOfDimensions=2  InputPortWidth=7  IndexOptions=Index vector (dialog),Index vector (dialog)  Indices=[1:3],[1:3]  OutputSizes=1
  Selector2 : Selector  InputPortWidth=2  IndexOptions=Index vector (dialog)  Indices=1  OutputSizes=1
  Selector3 : Selector  InputPortWidth=2  IndexOptions=Index vector (dialog)  Indices=2  OutputSizes=1
  Selector4 : Selector  InputPortWidth=2  IndexOptions=Index vector (dialog)  Indices=1  OutputSizes=1
  Selector5 : Selector  InputPortWidth=2  IndexOptions=Index vector (dialog)  Indices=2  OutputSizes=1
  Selector6 : Selector  InputPortWidth=2  IndexOptions=Index vector (dialog)  Indices=1  OutputSizes=1
  Selector7 : Selector  NumberOfDimensions=2  InputPortWidth=7  IndexOptions=Index vector (dialog),Index vector (dialog)  Indices=[1:3],[4]  OutputSizes=1
  Selector8 : Selector  NumberOfDimensions=2  InputPortWidth=7  IndexOptions=Index vector (dialog),Index vector (dialog)  Indices=[1:3],[1:3]  OutputSizes=1
  Selector9 : Selector  NumberOfDimensions=2  InputPortWidth=7  IndexOptions=Index vector (dialog),Index vector (dialog)  Indices=[1:3],[4]  OutputSizes=1
  Sqrt : Sqrt  Operator=signedSqrt  SaturateOnIntegerOverflow=on
  Subtract : Sum  Inputs=+-
  Switch : Switch  Criteria=u2 > Threshold
  one : Constant
  p_des_out : Outport  VectorParamsAs1DForOutWhenUnconnected=off
  dp_des_out : Outport  Port=2  VectorParamsAs1DForOutWhenUnconnected=off
  ddp_des_out : Outport  Port=3  VectorParamsAs1DForOutWhenUnconnected=off
  Euld_out : Outport  Port=4
  dEul_out : Outport  Port=5  VectorParamsAs1DForOutWhenUnconnected=off
  ddEul_out : Outport  Port=6  VectorParamsAs1DForOutWhenUnconnected=off
  trans_f : Outport  Port=7  VectorParamsAs1DForOutWhenUnconnected=off
  rot_f : Outport  Port=8  VectorParamsAs1DForOutWhenUnconnected=off
  wires:
  0_T_2/1 -> Reshape1/1
  0_T_1/1 -> Reshape/1
  Reshape/1 -> Selector7/1, Selector10/1
  Reshape1/1 -> Selector9/1, Selector8/1
  Product2/1 -> Angle Axis Via Quaternions/1(R)
  Angle Axis Via Quaternions/1(angle) -> rot_f/1
  Xd_in/1 -> Selector1/1, Selector2/1
  dXd_in/1 -> Selector4/1, Selector3/1
  ddXd_in/1 -> Selector6/1, Selector5/1
  Normalize/1(x/||x||) -> Product1/2, Product4/2, Product/2
  Selector5/1 -> Product1/1
  Selector3/1 -> Product4/1
  Selector1/1 -> Product/1
  Switch/1 -> Divide/1
  Product5/1 -> Add/1
  Abs1/1 -> trans_f/1, Switch/2, Switch/1
  Sqrt/1 -> Abs1/1
  Subtract/1 -> Dot Product/2, Dot Product/1, Divide/2
  Selector7/1 -> Add/2, Subtract/2
  one/1 -> Switch/3
  Selector9/1 -> Subtract/1
  Dot Product/1 -> Sqrt/1
  Divide/1 -> Product5/2, Product7/2, Product6/2
  Selector2/1 -> Product5/1
  Selector4/1 -> Product6/1
  Selector6/1 -> Product7/1
  Add/1 -> p_des_out/1
  Product6/1 -> dp_des_out/1
  Product7/1 -> ddp_des_out/1
  Product4/1 -> dEul_out/1
  Product1/1 -> ddEul_out/1
  Selector10/1 -> MATLAB Function/1(u), Product3/1, Math Function4/1
  Selector8/1 -> Product2/2
  Math Function4/1 -> Product2/1
  Product/1 -> Add1/2
  Product3/1 -> Normalize/1(x)
  Angle Axis Via Quaternions/2(axis) -> Product3/2
  MATLAB Function/1(y) -> Add1/1
  Add1/1 -> Euld_out/1

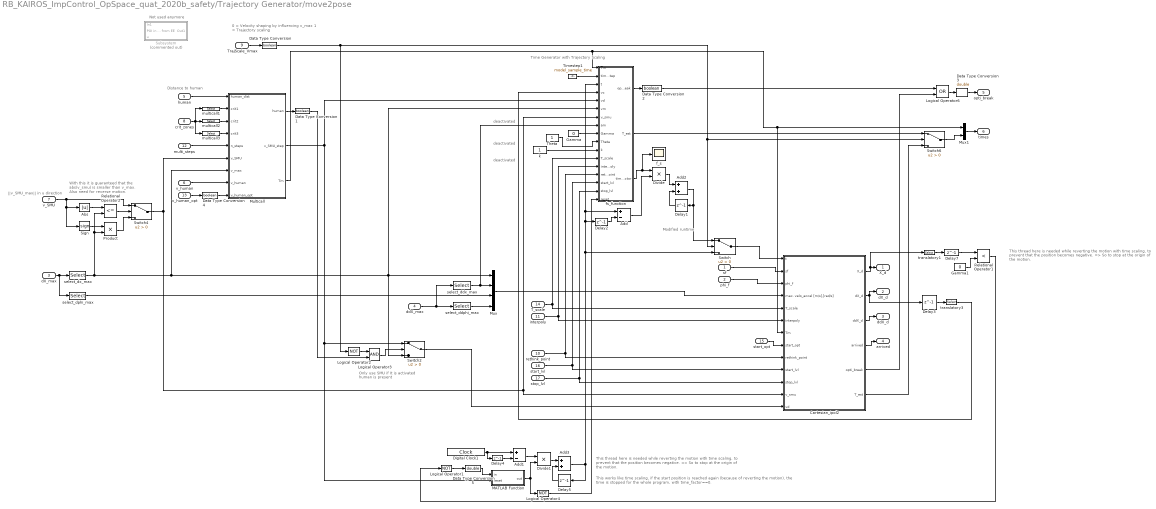
== system RB_KAIROS_ImpControl_OpSpace_quat_2020b_safety/Trajectory Generator/move2pose ==
  note: With this it is guaranteed that the
      | abs(v_smu) is smaller than v_max.
      | Also need for reverse motion.
  note: This works like time scaling, if the start position is reached again (because of reverting the motion),
      | the time is stopped for the whole program, with time_factor==0.
  note: This thread here is needed while reverting the motion with time scaling,
      | to prevent that the position becomes negative.
      | => So to stop at the origin of the motion.
  note: Distance to human
  note: 0 = Velocity shaping by influencing v_max
      | 1 = Trajectory scaling
  note: Only use SMU if
      | It is activated
      | human is present
  note: ||v_SMU_max|| in u direction
  note: Time Generator with Trajectory Scaling
  note: Modified runtime
  note: Not used anymore
  note: This thread here is needed while reverting the motion with time scaling,
      | to prevent that the position becomes negative.
      | => So to stop at the origin of the motion.
  note: deactivated
  note: deactivated
  note: deactivated
  sf : Inport
  phi_f : Inport  Port=2
  dX_max : Inport  Port=3
  ddX_max : Inport  Port=4
  human : Inport  Port=5
  v_human : Inport  Port=6
  v_SMU : Inport  Port=7
  crit_zones : Inport  Port=8
  TrajScale_Vmax : Inport  Port=9
  rethink_point : Inport  Port=10
  interpoly : Inport  Port=11
  multi_steps : Inport  Port=12
  v_human_opt : Inport  Port=13
  T_scale : Inport  Port=14
  start_opt : Inport  Port=15
  start_lvl : Inport  Port=16
  stop_lvl : Inport  Port=17
  Abs : Abs
  Add : Sum  Inputs=+-
  Add1 : Sum  Inputs=+-
  Add2 : Sum
  Add3 : Sum
  Cartesian_ipol2 : Subsystem  TreatAsAtomicUnit=on
  Data Type Conversion{,1..2,4} (4 alike) : DataTypeConversion  OutDataTypeStr=boolean
  Data Type Conversion3 : DataTypeConversion  OutDataTypeStr=double
  Data Type Conversion5 : DataTypeConversion  OutDataTypeStr=double
  Delay{1..5,7} (6 alike) : Delay  DelayLength=1
  Digital Clock1 : DigitalClock  SampleTime=model_sample_time
  Divide : Product  Inputs=**
  Divide1 : Product  Inputs=**
  Gamma : Constant  Value=0
  Gamma1 : Constant  Value=0
  Logical Operator1 : Logic  Operator=NOT  AllPortsSameDT=off  OutDataTypeStr=boolean
  Logical Operator2 : Logic  Operator=NOT  AllPortsSameDT=off  OutDataTypeStr=boolean
  Logical Operator3 : Logic  AllPortsSameDT=off  OutDataTypeStr=boolean
  Logical Operator4 : Logic  Operator=NOT  AllPortsSameDT=off  OutDataTypeStr=boolean
  Logical Operator6 : Logic  Operator=OR  AllPortsSameDT=off  OutDataTypeStr=boolean
  MATLAB Function : MATLAB Function  TreatAsAtomicUnit=on
  Multicall : MATLAB Function  TreatAsAtomicUnit=on
  Mux : Mux
  Mux1 : Mux  Inputs=2
  Product : Product
  Relational Operator1 : RelationalOperator  Operator=<  OutDataTypeStr=boolean  RndMeth=Simplest
  Relational Operator2 : RelationalOperator  Operator=<=  OutDataTypeStr=boolean  RndMeth=Simplest
  Sign : Signum
  Subsystem : Subsystem  Commented=on
  Switch{,2,4,6} (4 alike) : Switch  Criteria=u2 > Threshold
  Theta : Constant
  Timestep1 : Constant  Value=model_sample_time
  f_s : Scope
  fs_function : MATLAB Function  TreatAsAtomicUnit=on
  k : Constant
  multicall1 : Selector  InputPortWidth=3  IndexOptions=Index vector (dialog)  Indices=1  OutputSizes=1
  multicall2 : Selector  InputPortWidth=3  IndexOptions=Index vector (dialog)  Indices=2  OutputSizes=1
  multicall3 : Selector  InputPortWidth=3  IndexOptions=Index vector (dialog)  Indices=3  OutputSizes=1
  select_ddphi_max : Selector  InputPortWidth=2  IndexOptions=Index vector (dialog)  Indices=2  OutputSizes=1
  select_ddx_max : Selector  InputPortWidth=2  IndexOptions=Index vector (dialog)  Indices=1  OutputSizes=1
  select_dphi_max : Selector  InputPortWidth=2  IndexOptions=Index vector (dialog)  Indices=2  OutputSizes=1
  select_dx_max : Selector  InputPortWidth=2  IndexOptions=Index vector (dialog)  Indices=1  OutputSizes=1
  translatory1 : Selector  InputPortWidth=2  IndexOptions=Index vector (dialog)  Indices=1  OutputSizes=1
  translatory3 : Selector  InputPortWidth=2  IndexOptions=Index vector (dialog)  Indices=1  OutputSizes=1
  X_d : Outport  VectorParamsAs1DForOutWhenUnconnected=off
  dX_d : Outport  Port=2  VectorParamsAs1DForOutWhenUnconnected=off
  ddX_d : Outport  Port=3  VectorParamsAs1DForOutWhenUnconnected=off
  arrived : Outport  Port=4  VectorParamsAs1DForOutWhenUnconnected=off
  opti_break : Outport  Port=5  VectorParamsAs1DForOutWhenUnconnected=off
  times : Outport  Port=6  VectorParamsAs1DForOutWhenUnconnected=off
  wires:
  Switch4/1 -> Multicall/6(v_SMU), fs_function/7(v_smu), Cartesian_ipol2/12(v_smu)
  select_dphi_max/1 -> Mux/3
  multi_steps/1 -> Multicall/5(n_steps)
  interpoly/1 -> fs_function/13(interpoly), Cartesian_ipol2/6(interpoly)
  human/1 -> Multicall/1(human_dist)
  Logical Operator6/1 -> Data Type Conversion3/1
  Add2/1 -> Switch/1, Delay1/1
  Cartesian_ipol2/5(opti_break) -> Logical Operator6/2
  Multicall/3(Tm) -> fs_function/1(Tm), Cartesian_ipol2/7(Tm), Mux1/1
  Data Type Conversion2/1 -> Logical Operator6/1
  fs_function/1(opti_break) -> Data Type Conversion2/1
  Multicall/2(v_SMU_step) -> fs_function/5(vd), MATLAB Function/2(reset), Switch2/1
  Switch6/1 -> Mux1/2
  Cartesian_ipol2/2(dX_d) -> dX_d/1, Delay3/1
  Logical Operator3/1 -> Switch2/2
  Cartesian_ipol2/6(T_est) -> Switch6/3
  Mux1/1 -> times/1
  Theta/1 -> fs_function/10(Theta)
  select_dx_max/1 -> Multicall/7(v_max), fs_function/6(vm), Mux/1, Switch2/3, Product/2, Relational Operator2/2
  select_ddphi_max/1 -> Mux/4
  Divide/1 -> Add2/1
  fs_function/3(time_factor) -> f_s/1, Divide/1
  Data Type Conversion3/1 -> opti_break/1
  k/1 -> fs_function/11(k)
  crit_zones/1 -> multicall1/1, multicall2/1, multicall3/1
  Gamma/1 -> fs_function/9(Gamma)
  Mux/1 -> Cartesian_ipol2/4(max. velo_accel [m/s],[rad/s])
  select_ddx_max/1 -> fs_function/8(am), Mux/2
  Data Type Conversion/1 -> Logical Operator2/1, Switch6/2, Switch/2
  start_opt/1 -> Cartesian_ipol2/8(start_opt)
  TrajScale_Vmax/1 -> Data Type Conversion/1
  sf/1 -> Cartesian_ipol2/2(sf)
  Delay1/1 -> Add2/2
  Timestep1/1 -> fs_function/2(time_step)
  Delay3/1 -> translatory3/1
  stop_lvl/1 -> fs_function/16(stop_lvl), Cartesian_ipol2/11(stop_lvl)
  fs_function/2(T_est) -> Switch6/1
  dX_max/1 -> select_dphi_max/1, select_dx_max/1
  ddX_max/1 -> select_ddx_max/1, select_ddphi_max/1
  Cartesian_ipol2/4(arrived) -> arrived/1
  v_human/1 -> Multicall/8(v_human)
  Logical Operator2/1 -> Logical Operator3/1
  phi_f/1 -> Cartesian_ipol2/3(phi_f)
  rethink_point/1 -> fs_function/14(rethink_point), Cartesian_ipol2/9(rethink_point)
  Data Type Conversion1/1 -> Logical Operator3/2
  T_scale/1 -> fs_function/12(T_scale), Cartesian_ipol2/5(T_scale)
  start_lvl/1 -> fs_function/15(start_lvl), Cartesian_ipol2/10(start_lvl)
  Cartesian_ipol2/3(ddX_d) -> ddX_d/1
  translatory3/1 -> fs_function/4(vc)
  Add/1 -> Divide/2
  Switch/1 -> Cartesian_ipol2/1(t)
  Add3/1 -> Delay5/1, Add/1, fs_function/3(t), Delay2/1, Switch/3
  Delay2/1 -> Add/2
  Delay4/1 -> Add1/2
  Digital Clock1/1 -> Delay4/1, Add1/1
  Add1/1 -> Divide1/1
  Delay5/1 -> Add3/2
  Divide1/1 -> Add3/1
  translatory1/1 -> Delay7/1
  MATLAB Function/1(out) -> Divide1/2, Logical Operator4/1
  Logical Operator4/1 -> fs_function/17(reset)
  v_SMU/1 -> Sign/1, Abs/1, Switch4/1
  Relational Operator2/1 -> Switch4/2
  Abs/1 -> Relational Operator2/1
  Product/1 -> Switch4/3
  Sign/1 -> Product/1
  Switch2/1 -> Cartesian_ipol2/13(vd)
  Multicall/1(human) -> Data Type Conversion1/1
  multicall1/1 -> Multicall/2(crit1)
  multicall2/1 -> Multicall/3(crit2)
  multicall3/1 -> Multicall/4(crit3)
  v_human_opt/1 -> Data Type Conversion4/1
  Data Type Conversion4/1 -> Multicall/9(v_human_opt)
  Cartesian_ipol2/1(X_d) -> translatory1/1, X_d/1
  Delay7/1 -> Relational Operator1/1
  Gamma1/1 -> Relational Operator1/2
  Relational Operator1/1 -> Logical Operator1/1
  Data Type Conversion5/1 -> MATLAB Function/1(in)
  Logical Operator1/1 -> Data Type Conversion5/1

== system RB_KAIROS_ImpControl_OpSpace_quat_2020b_safety/CONTROLLER /Kinematics and Dynamics/Dynamics - Configuration space ==
  qv : Inport
  qa : Inport  Port=2
  "qv_dot " : Inport  Port=3
  qa_dot : Inport  Port=4
  "Arm Coriolis/Centrifugal Matrix " : MATLAB Function  TreatAsAtomicUnit=on
  Arm Gravity terms : MATLAB Function  TreatAsAtomicUnit=on
  "Chassis Coriolis/Centrifugal Matrix " : MATLAB Function  TreatAsAtomicUnit=on
  Chassis Mass Matrix : MATLAB Function  TreatAsAtomicUnit=on
  Gravitational acceleration : Constant  Value=9.8067
  MATLAB Function : MATLAB Function  TreatAsAtomicUnit=on
  MATLAB Function1 : MATLAB Function  TreatAsAtomicUnit=on
  MATLAB Function4 : MATLAB Function  TreatAsAtomicUnit=on
  M : Outport
  C : Outport  Port=2
  G : Outport  Port=3
  wires:
  Arm Gravity terms/1(G) -> G/1
  Gravitational acceleration/1 -> Arm Gravity terms/3(g)
  MATLAB Function1/1(C) -> C/1
  qa/1 -> "Arm Coriolis/Centrifugal Matrix "/2(qa), Arm Gravity terms/2(qa), MATLAB Function4/2(qa)
  "Arm Coriolis/Centrifugal Matrix "/1(C) -> MATLAB Function1/1(C_a)
  qa_dot/1 -> "Arm Coriolis/Centrifugal Matrix "/4(qda)
  qv/1 -> "Chassis Coriolis/Centrifugal Matrix "/1(qv), Arm Gravity terms/1(qv), "Arm Coriolis/Centrifugal Matrix "/1(qv), Chassis Mass Matrix/1(qv), MATLAB Function4/1(qv)
  "Chassis Coriolis/Centrifugal Matrix "/1(Cv) -> MATLAB Function1/2(C_v)
  "qv_dot "/1 -> "Arm Coriolis/Centrifugal Matrix "/3(qdv), "Chassis Coriolis/Centrifugal Matrix "/2(qdv)
  MATLAB Function4/1(M) -> MATLAB Function/1(M_a)
  Chassis Mass Matrix/1(Mv) -> MATLAB Function/2(M_v)
  MATLAB Function/1(M) -> M/1
